simulink model "Induction_motor_with_three_phase_vsi_without_pwm_technique"  (R2014a)
settings: Solver=ode23t  StartTime=0.0  StopTime=1  MaxStep=1e-6  RelTol=1e-3
libraries: powerlib x12, powerlib_meascontrol x2
settings Model: Creator=singa  LastModifiedBy=singa

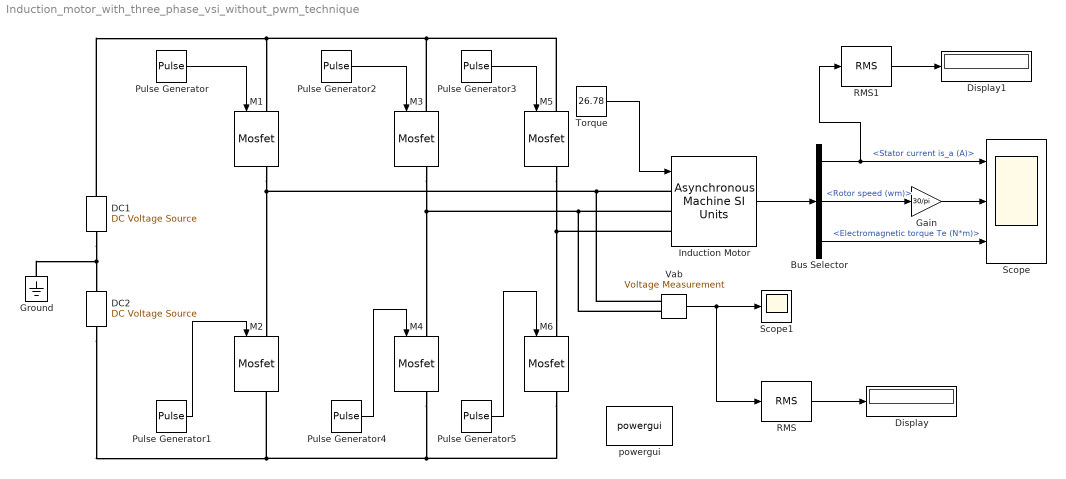
== system Induction_motor_with_three_phase_vsi_without_pwm_technique ==
  Bus Selector : BusSelector  OutputSignals=Stator measurements.Stator current is_a (A),Mechanical.Rotor speed (wm),Mechanical.Electromagnetic torque Te (N*m)
  DC1 : powerlib/Electrical Sources/DC Voltage Source  Amplitude=257  Measurements=None
  DC2 : powerlib/Electrical Sources/DC Voltage Source  Amplitude=257  Measurements=None
  Display : Display
  Display1 : Display
  Gain : Gain  Gain=30/pi
  Ground : powerlib/Elements/Ground  LConnTagsString=a
  Induction Motor : powerlib/Machines/Asynchronous Machine SI Units  PresetModel="15:  5.4 HP (4KW)   400 V  50Hz 1430 RPM"  MechanicalLoad=Torque Tm  ShowDetailedParameters=on  RotorType=Squirrel-cage  ReferenceFrame=Rotor  Units=SI  MeasurementBus=off  NominalParameters=[4000 400 50]  Stator=[1.405 0.005839]  Rotor=[1.395 0.005839]  Cage1=[ 0.022 0.226/377]  Cage2=[ 0.022 0.226/377]  Lm=0.1722  Mechanical=[0.0131 0.002985 2]  PolePairs=2  InitialConditions=[1 0 0 0 0 0 0 0]  SimulateSaturation=off  Saturation=[14.03593122, 27.81365428, 53.79336849, 72.68890987, 97.98006896, 148.6815601, 215.7428561, 302.9841135, 420.4778367 ; 230, 322, 414, 460, 506, 552, 598, 644, 690]  LoadFlowParameters=1492000  TsPowergui=0  TsBlock=-1  IterativeModel=Trapezoidal non iterative  Pmec=0
  M{1..6} (6 alike) : powerlib/Power Electronics/Mosfet  Ron=0.1  Lon=0  Rd=0.01  Vfd=0  IC=0  Rs=1e5  Cs=inf  Measurements=on
  Pulse Generator : DiscretePulseGenerator  PulseType=Time based  Period=0.02  PulseWidth=50
  Pulse Generator1 : DiscretePulseGenerator  PulseType=Time based  Period=0.02  PulseWidth=50  PhaseDelay=0.01
  Pulse Generator2 : DiscretePulseGenerator  PulseType=Time based  Period=0.02  PulseWidth=50  PhaseDelay=0.02/3
  Pulse Generator3 : DiscretePulseGenerator  PulseType=Time based  Period=0.02  PulseWidth=50  PhaseDelay=0.04/3
  Pulse Generator4 : DiscretePulseGenerator  PulseType=Time based  Period=0.02  PulseWidth=50  PhaseDelay=0.01+0.02/3
  Pulse Generator5 : DiscretePulseGenerator  PulseType=Time based  Period=0.02  PulseWidth=50  PhaseDelay=0.01+0.04/3
  RMS : powerlib_meascontrol/Measurements/RMS  TrueRMS=on  Freq=50  RMSInit=120  Ts=0
  RMS1 : powerlib_meascontrol/Measurements/RMS  TrueRMS=on  Freq=50  RMSInit=120  Ts=0
  Scope : Scope  NumInputPorts=3
      settings: YMin=-5~-5~-5  YMax=5~5~5  SampleInput=on  SampleTime=1e-6
  Scope1 : Scope
      settings: SampleInput=on  SampleTime=1e-6
  Torque : Constant  Value=26.78
  Vab : powerlib/Measurements/Voltage Measurement  PhasorSimulation=off  OutputType=Complex  PSBequivalent=0
  powergui : powerlib/powergui  Priority=1  SimulationMode=Continuous  SolverType=Tustin  SampleTime=50e-6  frequency=60  SPID=off  DisableSnubberDevices=off  DisableRonSwitches=off  DisableVfSwitches=off  SwTol=0  Interpol=off  DisplayEquations=off  Ts=0  methode=off  frequencyindice=50  Pbase=100e6  ErrMax=1e-4  Iterations=50  UnitsV=kV  UnitsW=MW  FunctionMessages=off  echomessages=off  HookPort=off  EnableUseOfTLC=off  x0status=blocks  RestoreLinks=warning  ResistiveCurrentMeasurement=off  Frange=[0:2:500]  Ylog=off  Xlog=on  ShowGrid=off  save=off  variable=ZData  structure=ScopeData1  ZoomFFT=off  StartTime=0.5  cycles=2  DisplayStyle=4  fundamental=50  FreqAxis=on  MaxFrequency=2500  frequencyindicesteady=1  RmsSteady=1  display=off
  wires:
  Pulse Generator/1 -> M1/1
  Pulse Generator1/1 -> M2/1
  Pulse Generator2/1 -> M3/1
  Pulse Generator3/1 -> M5/1
  Pulse Generator4/1 -> M4/1
  Pulse Generator5/1 -> M6/1
  Induction Motor/1 -> Bus Selector/1
  Bus Selector/1 -> RMS1/1, Scope/1  "<Stator current is_a (A)>"
  Bus Selector/3 -> Scope/3  "<Electromagnetic torque Te (N*m)>"
  Torque/1 -> Induction Motor/1
  Bus Selector/2 -> Gain/1  "<Rotor speed (wm)>"
  Gain/1 -> Scope/2
  Vab/1 -> RMS/1, Scope1/1
  RMS/1 -> Display/1
  RMS1/1 -> Display1/1
  connections:
  DC1/LConn1 -- Ground/LConn1 -- DC2/RConn1
  DC1/RConn1 -- M5/LConn1 -- M3/LConn1 -- M1/LConn1
  DC2/LConn1 -- M6/RConn1 -- M4/RConn1 -- M2/RConn1
  M5/RConn1 -- Induction Motor/LConn3 -- M6/LConn1
  M3/RConn1 -- Vab/LConn2 -- Induction Motor/LConn2 -- M4/LConn1
  M1/RConn1 -- Vab/LConn1 -- Induction Motor/LConn1 -- M2/LConn1
